simulink model "FSAC2021_V1_Running"  (R2014a)
settings: Solver=FixedStepDiscrete  StartTime=0.0  StopTime=inf  FixedStep=0.0005  RelTol=1e-3
model workspace (MAT data in the model file):
  MCOS : class17 (value not decoded)
  MCOS : class17 (value not decoded)
  MCOS : class17 (value not decoded)
  MCOS : class17 (value not decoded)
  MCOS : class17 (value not decoded)
  MCOS : class17 (value not decoded)
  MCOS : class17 (value not decoded)
  MCOS : class17 (value not decoded)
  MCOS : class17 (value not decoded)
  MCOS : class17 (value not decoded)
  MCOS : class17 (value not decoded)
  MCOS : class17 (value not decoded)
  MCOS : class17 (value not decoded)
  MCOS : class17 (value not decoded)
  MCOS : class17 (value not decoded)
  MCOS : class17 (value not decoded)
  MCOS : class17 (value not decoded)
  MCOS : class17 (value not decoded)
  MCOS : class17 (value not decoded)
  BUZZER_START = 1
  MCOS : class17 (value not decoded)
  MCOS : class17 (value not decoded)
  MCOS : class17 (value not decoded)
  MCOS : class17 (value not decoded)
  MCOS : class17 (value not decoded)
  MCOS : class17 (value not decoded)
  MCOS : class17 (value not decoded)
  MCOS : class17 (value not decoded)
  MCOS : class17 (value not decoded)
  MCOS : class17 (value not decoded)
  MCOS : class17 (value not decoded)
  MCOS : class17 (value not decoded)
  MCOS : class17 (value not decoded)
  MCOS : class17 (value not decoded)
  MCOS : class17 (value not decoded)
  MCOS : class17 (value not decoded)
  MCOS : class17 (value not decoded)
  MCOS : class17 (value not decoded)
  MCOS : class17 (value not decoded)
  MCOS : class17 (value not decoded)
  MCOS : class17 (value not decoded)
  MCOS : class17 (value not decoded)
  MCOS : class17 (value not decoded)
  MCOS : class17 (value not decoded)
  MCOS : class17 (value not decoded)
  MCOS : class17 (value not decoded)
  MCOS : class17 (value not decoded)
  MCOS : class17 (value not decoded)
  MCOS : class17 (value not decoded)
  MCOS : class17 (value not decoded)
  MCOS : class17 (value not decoded)
  MCOS : class17 (value not decoded)
  MCOS : class17 (value not decoded)
  MCOS : class17 (value not decoded)
  MCOS : class17 (value not decoded)
  MCOS : class17 (value not decoded)
  MCOS : class17 (value not decoded)
  MCOS : class17 (value not decoded)
  Brake = 11
  MCOS : class17 (value not decoded)
  MCOS : class17 (value not decoded)
  MCOS : class17 (value not decoded)
  MCOS : class17 (value not decoded)
  MCOS : class17 (value not decoded)
  MCOS : class17 (value not decoded)
  MCOS : class17 (value not decoded)
  MCOS : class17 (value not decoded)
  Sensor_Acc_b = 101.85
  Sensor_Acc_k = -0.0185
  Str_Sen_Orig_Angle = -341
  MCOS : class17 (value not decoded)
  Tire_D = 0.47
  T = 0.05
libraries: simulink x402, ec55xxlib x134
(part 7 of 17)

== system FSAC2021_V1_Running/VCU_CAN_Read/PCANB(BMS、DRIVE_MOTOR)/BMS_HCU_MAXT1 ==
  input : Inport
  function : TriggerPort  TriggerType=function-call
  CoolingCtl_Ad : Sum
  CoolingCtl_Convert : DataTypeConversion  OutDataTypeStr=uint32
  CoolingCtl_F : Gain
  CoolingCtl_L : simulink/Logic and Bit Operations/Bitwise Operator  logicop=AND  UseBitMask=on  BitMask=255  BitMaskRealWorld=Stored Integer
  CoolingCtl_O : Constant  Value=0  OutDataTypeStr=single
  CoolingCtl_S : ArithShift
  CoolingCtl_Sub : Subsystem
  CoolingCtl_sat : Saturate  UpperLimit=1  LowerLimit=0
  CoolingCtlcv : DataTypeConversion
  Demux : Demux  Outputs=8
  HeatingCtl_Ad : Sum
  HeatingCtl_Convert : DataTypeConversion  OutDataTypeStr=uint32
  HeatingCtl_F : Gain
  HeatingCtl_L : simulink/Logic and Bit Operations/Bitwise Operator  logicop=AND  UseBitMask=on  BitMask=255  BitMaskRealWorld=Stored Integer
  HeatingCtl_O : Constant  Value=0  OutDataTypeStr=single
  HeatingCtl_S : ArithShift
  HeatingCtl_Sub : Subsystem
  HeatingCtl_sat : Saturate  UpperLimit=1  LowerLimit=0
  HeatingCtlcv : DataTypeConversion
  MaxTempNo_Ad : Sum
  MaxTempNo_Convert : DataTypeConversion  OutDataTypeStr=uint32
  MaxTempNo_F : Gain
  MaxTempNo_L : simulink/Logic and Bit Operations/Bitwise Operator  logicop=AND  UseBitMask=on  BitMask=255  BitMaskRealWorld=Stored Integer
  MaxTempNo_O : Constant  Value=0  OutDataTypeStr=single
  MaxTempNo_S : ArithShift
  MaxTempNo_Sub : Subsystem
  MaxTempNo_sat : Saturate  UpperLimit=255  LowerLimit=0
  MaxTempNocv : DataTypeConversion
  MaxTemp_Ad : Sum
  MaxTemp_Convert : DataTypeConversion  OutDataTypeStr=uint32
  MaxTemp_F : Gain
  MaxTemp_L : simulink/Logic and Bit Operations/Bitwise Operator  logicop=AND  UseBitMask=on  BitMask=255  BitMaskRealWorld=Stored Integer
  MaxTemp_O : Constant  Value=-40  OutDataTypeStr=single
  MaxTemp_S : ArithShift
  MaxTemp_Sub : Subsystem
  MaxTemp_sat : Saturate  UpperLimit=120  LowerLimit=-40
  MaxTempcv : DataTypeConversion
  MinTempNo_Ad : Sum
  MinTempNo_Convert : DataTypeConversion  OutDataTypeStr=uint32
  MinTempNo_F : Gain
  MinTempNo_L : simulink/Logic and Bit Operations/Bitwise Operator  logicop=AND  UseBitMask=on  BitMask=255  BitMaskRealWorld=Stored Integer
  MinTempNo_O : Constant  Value=0  OutDataTypeStr=single
  MinTempNo_S : ArithShift
  MinTempNo_Sub : Subsystem
  MinTempNo_sat : Saturate  UpperLimit=255  LowerLimit=0
  MinTempNocv : DataTypeConversion
  MinTemp_Ad : Sum
  MinTemp_Convert : DataTypeConversion  OutDataTypeStr=uint32
  MinTemp_F : Gain
  MinTemp_L : simulink/Logic and Bit Operations/Bitwise Operator  logicop=AND  UseBitMask=on  BitMask=255  BitMaskRealWorld=Stored Integer
  MinTemp_O : Constant  Value=-40  OutDataTypeStr=single
  MinTemp_S : ArithShift
  MinTemp_Sub : Subsystem
  MinTemp_sat : Saturate  UpperLimit=120  LowerLimit=-40
  MinTempcv : DataTypeConversion
  HeatingCtl_Out : Outport
  CoolingCtl_Out : Outport  Port=2
  MinTempNo_Out : Outport  Port=3
  MaxTempNo_Out : Outport  Port=4
  MinTemp_Out : Outport  Port=5
  MaxTemp_Out : Outport  Port=6
  wires:
  HeatingCtl_F/1 -> HeatingCtl_Ad/1
  HeatingCtl_O/1 -> HeatingCtl_Ad/2
  HeatingCtl_Ad/1 -> HeatingCtl_sat/1
  HeatingCtl_sat/1 -> HeatingCtl_Out/1
  Demux/6 -> HeatingCtl_Sub/1(In1)
  HeatingCtl_Sub/1(Out1) -> HeatingCtl_Convert/1
  HeatingCtl_Convert/1 -> HeatingCtl_L/1
  HeatingCtl_L/1 -> HeatingCtl_S/1
  HeatingCtl_S/1 -> HeatingCtlcv/1
  HeatingCtlcv/1 -> HeatingCtl_F/1
  CoolingCtl_F/1 -> CoolingCtl_Ad/1
  CoolingCtl_O/1 -> CoolingCtl_Ad/2
  CoolingCtl_Ad/1 -> CoolingCtl_sat/1
  CoolingCtl_sat/1 -> CoolingCtl_Out/1
  Demux/5 -> CoolingCtl_Sub/1(In1)
  CoolingCtl_Sub/1(Out1) -> CoolingCtl_Convert/1
  CoolingCtl_Convert/1 -> CoolingCtl_L/1
  CoolingCtl_L/1 -> CoolingCtl_S/1
  CoolingCtl_S/1 -> CoolingCtlcv/1
  CoolingCtlcv/1 -> CoolingCtl_F/1
  MinTempNo_F/1 -> MinTempNo_Ad/1
  MinTempNo_O/1 -> MinTempNo_Ad/2
  MinTempNo_Ad/1 -> MinTempNo_sat/1
  MinTempNo_sat/1 -> MinTempNo_Out/1
  Demux/4 -> MinTempNo_Sub/1(In1)
  MinTempNo_Sub/1(Out1) -> MinTempNo_Convert/1
  MinTempNo_Convert/1 -> MinTempNo_L/1
  MinTempNo_L/1 -> MinTempNo_S/1
  MinTempNo_S/1 -> MinTempNocv/1
  MinTempNocv/1 -> MinTempNo_F/1
  MaxTempNo_F/1 -> MaxTempNo_Ad/1
  MaxTempNo_O/1 -> MaxTempNo_Ad/2
  MaxTempNo_Ad/1 -> MaxTempNo_sat/1
  MaxTempNo_sat/1 -> MaxTempNo_Out/1
  Demux/3 -> MaxTempNo_Sub/1(In1)
  MaxTempNo_Sub/1(Out1) -> MaxTempNo_Convert/1
  MaxTempNo_Convert/1 -> MaxTempNo_L/1
  MaxTempNo_L/1 -> MaxTempNo_S/1
  MaxTempNo_S/1 -> MaxTempNocv/1
  MaxTempNocv/1 -> MaxTempNo_F/1
  MinTemp_F/1 -> MinTemp_Ad/1
  MinTemp_O/1 -> MinTemp_Ad/2
  MinTemp_Ad/1 -> MinTemp_sat/1
  MinTemp_sat/1 -> MinTemp_Out/1
  Demux/2 -> MinTemp_Sub/1(In1)
  MinTemp_Sub/1(Out1) -> MinTemp_Convert/1
  MinTemp_Convert/1 -> MinTemp_L/1
  MinTemp_L/1 -> MinTemp_S/1
  MinTemp_S/1 -> MinTempcv/1
  MinTempcv/1 -> MinTemp_F/1
  MaxTemp_F/1 -> MaxTemp_Ad/1
  MaxTemp_O/1 -> MaxTemp_Ad/2
  MaxTemp_Ad/1 -> MaxTemp_sat/1
  MaxTemp_sat/1 -> MaxTemp_Out/1
  Demux/1 -> MaxTemp_Sub/1(In1)
  MaxTemp_Sub/1(Out1) -> MaxTemp_Convert/1
  MaxTemp_Convert/1 -> MaxTemp_L/1
  MaxTemp_L/1 -> MaxTemp_S/1
  MaxTemp_S/1 -> MaxTempcv/1
  MaxTempcv/1 -> MaxTemp_F/1
  input/1 -> Demux/1

== system FSAC2021_V1_Running/VCU_CAN_Read/PCANB(BMS、DRIVE_MOTOR)/BMS_HCU_MAXV  ==
  In1 : Inport
  function : TriggerPort  TriggerType=function-call
  BMS_HCU_MAXV : Subsystem
  Data Type Conversion{8..11} (4 alike) : DataTypeConversion  OutDataTypeStr=uint16
  MaxCellVoltNo_Out : Outport
  MinCellVoltNo_Out : Outport  Port=2
  MinCellVolt_Out : Outport  Port=3
  MaxCellVolt_Out : Outport  Port=4
  wires:
  BMS_HCU_MAXV/3(MinCellVolt_Out) -> Data Type Conversion10/1
  BMS_HCU_MAXV/4(MaxCellVolt_Out) -> Data Type Conversion11/1
  BMS_HCU_MAXV/1(MaxCellVoltNo_Out) -> Data Type Conversion8/1
  BMS_HCU_MAXV/2(MinCellVoltNo_Out) -> Data Type Conversion9/1
  Data Type Conversion8/1 -> MaxCellVoltNo_Out/1
  Data Type Conversion9/1 -> MinCellVoltNo_Out/1
  Data Type Conversion10/1 -> MinCellVolt_Out/1
  Data Type Conversion11/1 -> MaxCellVolt_Out/1
  In1/1 -> BMS_HCU_MAXV/1(input)

== system FSAC2021_V1_Running/VCU_CAN_Read/PCANB(BMS、DRIVE_MOTOR)/BMS_HCU_POWER  ==
  In1 : Inport
  function : TriggerPort  TriggerType=function-call
  BMS_HCU_POWER : Subsystem
  Data Type Conversion{74..77} (4 alike) : DataTypeConversion  OutDataTypeStr=double
  MaxDisPowerLimit_Out : Outport
  MaxChrPowerLimit_Out : Outport  Port=2
  MaxDisCurtLimit_Out : Outport  Port=3
  MaxChrCurtLimit_Out : Outport  Port=4
  wires:
  Data Type Conversion75/1 -> MaxChrPowerLimit_Out/1
  Data Type Conversion74/1 -> MaxDisPowerLimit_Out/1
  Data Type Conversion76/1 -> MaxDisCurtLimit_Out/1
  Data Type Conversion77/1 -> MaxChrCurtLimit_Out/1
  BMS_HCU_POWER/2(MaxChrPowerLimit_Out) -> Data Type Conversion75/1
  BMS_HCU_POWER/3(MaxDisCurtLimit_Out) -> Data Type Conversion76/1
  BMS_HCU_POWER/4(MaxChrCurtLimit_Out) -> Data Type Conversion77/1
  BMS_HCU_POWER/1(MaxDisPowerLimit_Out) -> Data Type Conversion74/1
  In1/1 -> BMS_HCU_POWER/1(input)

== system FSAC2021_V1_Running/VCU_CAN_Read/PCANB(BMS、DRIVE_MOTOR)/BMS_RELAY  ==
  In1 : Inport
  function : TriggerPort  TriggerType=function-call
  BMS_HCU_RELAY : Subsystem
  Data Type Conversion{63,66..73} (9 alike) : DataTypeConversion  OutDataTypeStr=uint8
  Data Type Conversion64 : DataTypeConversion  OutDataTypeStr=double
  Data Type Conversion65 : DataTypeConversion  OutDataTypeStr=double
  offChrRlyStr_Out : Outport
  ChrReqCurr_Out : Outport  Port=2
  ChrReqVolt_Out : Outport  Port=3
  chrONCC_Out : Outport  Port=4
  chrOFFCC2_Out : Outport  Port=5
  ChrCommunication_Out : Outport  Port=6
  ChrState_Out : Outport  Port=7
  OnChrRlyStr_Out : Outport  Port=8
  PreRlyStr_Out : Outport  Port=9
  NegRlyStr_Out : Outport  Port=10
  PosRlyStr_Out : Outport  Port=11
  wires:
  Data Type Conversion67/1 -> chrOFFCC2_Out/1
  Data Type Conversion63/1 -> offChrRlyStr_Out/1
  Data Type Conversion64/1 -> ChrReqCurr_Out/1
  Data Type Conversion69/1 -> ChrState_Out/1
  Data Type Conversion71/1 -> PreRlyStr_Out/1
  Data Type Conversion65/1 -> ChrReqVolt_Out/1
  Data Type Conversion73/1 -> PosRlyStr_Out/1
  Data Type Conversion72/1 -> NegRlyStr_Out/1
  Data Type Conversion66/1 -> chrONCC_Out/1
  Data Type Conversion68/1 -> ChrCommunication_Out/1
  Data Type Conversion70/1 -> OnChrRlyStr_Out/1
  BMS_HCU_RELAY/1(offChrRlyStr_Out) -> Data Type Conversion63/1
  BMS_HCU_RELAY/2(ChrReqCurr_Out) -> Data Type Conversion64/1
  BMS_HCU_RELAY/4(chrONCC_Out) -> Data Type Conversion66/1
  BMS_HCU_RELAY/9(PreRlyStr_Out) -> Data Type Conversion71/1
  BMS_HCU_RELAY/11(PosRlyStr_Out) -> Data Type Conversion73/1
  BMS_HCU_RELAY/8(OnChrRlyStr_Out) -> Data Type Conversion70/1
  BMS_HCU_RELAY/5(chrOFFCC2_Out) -> Data Type Conversion67/1
  BMS_HCU_RELAY/10(NegRlyStr_Out) -> Data Type Conversion72/1
  BMS_HCU_RELAY/6(ChrCommunication_Out) -> Data Type Conversion68/1
  BMS_HCU_RELAY/3(ChrReqVolt_Out) -> Data Type Conversion65/1
  BMS_HCU_RELAY/7(ChrState_Out) -> Data Type Conversion69/1
  In1/1 -> BMS_HCU_RELAY/1(input)

== system FSAC2021_V1_Running/VCU_CAN_Read/PCANB(BMS、DRIVE_MOTOR)/MOTOR_CURRENT_SPEED ==
  input : Inport
  function : TriggerPort  TriggerType=function-call
  Demux : Demux  Outputs=2
  Motor_Currt_Speed_Ad : Sum
  Motor_Currt_Speed_Convert : DataTypeConversion  OutDataTypeStr=uint32
  Motor_Currt_Speed_F : Gain
  Motor_Currt_Speed_L : simulink/Logic and Bit Operations/Bitwise Operator  logicop=AND  UseBitMask=on  BitMask=65535  BitMaskRealWorld=Stored Integer
  Motor_Currt_Speed_O : Constant  Value=0  OutDataTypeStr=single
  Motor_Currt_Speed_S : ArithShift
  Motor_Currt_Speed_Sub : Subsystem
  Motor_Currt_Speed_sat : Saturate  UpperLimit=2500  LowerLimit=0
  Motor_Currt_Speedcv : DataTypeConversion
  Motor_Currt_Speedinput2_Ad : Sum
  Motor_Currt_Speedinput2_C : Constant  Value=256
  Motor_Currt_Speedinput2_P : Product
  Motor_Currt_Speed_Out : Outport
  wires:
  Motor_Currt_Speed_F/1 -> Motor_Currt_Speed_Ad/1
  Motor_Currt_Speed_O/1 -> Motor_Currt_Speed_Ad/2
  Motor_Currt_Speed_Ad/1 -> Motor_Currt_Speed_sat/1
  Motor_Currt_Speed_sat/1 -> Motor_Currt_Speed_Out/1
  Demux/2 -> Motor_Currt_Speedinput2_P/1
  Motor_Currt_Speedinput2_C/1 -> Motor_Currt_Speedinput2_P/2
  Motor_Currt_Speedinput2_P/1 -> Motor_Currt_Speedinput2_Ad/1
  Demux/1 -> Motor_Currt_Speedinput2_Ad/2
  Motor_Currt_Speedinput2_Ad/1 -> Motor_Currt_Speed_Sub/1(In1)
  Motor_Currt_Speed_Sub/1(Out1) -> Motor_Currt_Speed_Convert/1
  Motor_Currt_Speed_Convert/1 -> Motor_Currt_Speed_L/1
  Motor_Currt_Speed_L/1 -> Motor_Currt_Speed_S/1
  Motor_Currt_Speed_S/1 -> Motor_Currt_Speedcv/1
  Motor_Currt_Speedcv/1 -> Motor_Currt_Speed_F/1
  input/1 -> Demux/1

== system FSAC2021_V1_Running/VCU_CAN_Read/Subsystem/BMS_HCU_INFO  ==
  In1 : Inport
  function : TriggerPort  TriggerType=function-call
  BMS_HCU_INFO : Subsystem
  Data Type Conversion{78..82} (5 alike) : DataTypeConversion  OutDataTypeStr=uint8
  Data Type Conversion83 : DataTypeConversion  OutDataTypeStr=double
  Data Type Conversion84 : DataTypeConversion  OutDataTypeStr=double
  BatLife_Out : Outport
  BatAlmLv_Out : Outport  Port=2
  BatState_Out : Outport  Port=3
  BatSoh_Out : Outport  Port=4
  BatSoc_Out : Outport  Port=5
  BatCurrent_Out : Outport  Port=6
  BatVoltage_Out : Outport  Port=7
  wires:
  Data Type Conversion79/1 -> BatAlmLv_Out/1
  Data Type Conversion80/1 -> BatState_Out/1
  Data Type Conversion84/1 -> BatVoltage_Out/1
  Data Type Conversion82/1 -> BatSoc_Out/1
  Data Type Conversion78/1 -> BatLife_Out/1
  Data Type Conversion81/1 -> BatSoh_Out/1
  Data Type Conversion83/1 -> BatCurrent_Out/1
  BMS_HCU_INFO/3(BatState_Out) -> Data Type Conversion80/1
  BMS_HCU_INFO/6(BatCurrent_Out) -> Data Type Conversion83/1
  BMS_HCU_INFO/4(BatSoh_Out) -> Data Type Conversion81/1
  BMS_HCU_INFO/5(BatSoc_Out) -> Data Type Conversion82/1
  BMS_HCU_INFO/7(BatVoltage_Out) -> Data Type Conversion84/1
  BMS_HCU_INFO/1(BatLife_Out) -> Data Type Conversion78/1
  BMS_HCU_INFO/2(BatAlmLv_Out) -> Data Type Conversion79/1
  In1/1 -> BMS_HCU_INFO/1(input)

== system FSAC2021_V1_Running/VCU_CAN_Read/Subsystem1/HEARTBEAT  ==
  In1 : Inport
  function : TriggerPort  TriggerType=function-call
  Data Type Conversion21 : DataTypeConversion  OutDataTypeStr=uint8
  MOTEC_HEARTBEAT : Subsystem
  Heartbeat_info_Out : Outport
  wires:
  MOTEC_HEARTBEAT/1(Heartbeat_info_Out) -> Data Type Conversion21/1
  Data Type Conversion21/1 -> Heartbeat_info_Out/1
  In1/1 -> MOTEC_HEARTBEAT/1(input)

== system FSAC2021_V1_Running/VCU_CAN_Read/Subsystem2/MOTEC_STATUS  ==
  In1 : Inport
  function : TriggerPort  TriggerType=function-call
  Data Type Conversion{13,15..20,106..107} (9 alike) : DataTypeConversion  OutDataTypeStr=uint8
  MOTEC_STATUS : Subsystem
  Fault_Out : Outport
  Operation_Enabled_Out : Outport  Port=2
  Quick_Stop_Out : Outport  Port=3
  Ready_Switch_On_Out : Outport  Port=4
  Switch_On_Disabled_Out : Outport  Port=5
  Swtiched_On_Out : Outport  Port=6
  Target_Reached_Out : Outport  Port=7
  Voltage_Enabled_Out : Outport  Port=8
  Warning_Out : Outport  Port=9
  wires:
  In1/1 -> MOTEC_STATUS/1(input)
  MOTEC_STATUS/3(Quick_Stop_Out) -> Data Type Conversion16/1
  MOTEC_STATUS/4(Ready_Switch_On_Out) -> Data Type Conversion17/1
  MOTEC_STATUS/5(Switch_On_Disabled_Out) -> Data Type Conversion18/1
  MOTEC_STATUS/6(Swtiched_On_Out) -> Data Type Conversion19/1
  MOTEC_STATUS/1(Fault_Out) -> Data Type Conversion13/1
  MOTEC_STATUS/2(Operation_Enabled_Out) -> Data Type Conversion15/1
  Data Type Conversion15/1 -> Operation_Enabled_Out/1
  Data Type Conversion17/1 -> Ready_Switch_On_Out/1
  Data Type Conversion20/1 -> Target_Reached_Out/1
  Data Type Conversion19/1 -> Swtiched_On_Out/1
  Data Type Conversion16/1 -> Quick_Stop_Out/1
  Data Type Conversion18/1 -> Switch_On_Disabled_Out/1
  MOTEC_STATUS/8(Voltage_Enabled_Out) -> Data Type Conversion106/1
  Data Type Conversion107/1 -> Warning_Out/1
  MOTEC_STATUS/7(Target_Reached_Out) -> Data Type Conversion20/1
  MOTEC_STATUS/9(Warning_Out) -> Data Type Conversion107/1
  Data Type Conversion106/1 -> Voltage_Enabled_Out/1
  Data Type Conversion13/1 -> Fault_Out/1

== system FSAC2021_V1_Running/CAN_SEND/(BRK、STR、DRIVER)/BCU_MTR_MOVE_AB/Brake_mtr_goalpos ==
  Brake_mtr_goalpos : Inport
  Brake_mtr_goalposABS : Abs
  Brake_mtr_goalposBitCov : DataTypeConversion  OutDataTypeStr=uint32
  Brake_mtr_goalposBitCov1 : DataTypeConversion  OutDataTypeStr=uint32
  Brake_mtr_goalposBitCov2 : DataTypeConversion  OutDataTypeStr=uint8
  Brake_mtr_goalposCOV : DataTypeConversion  OutDataTypeStr=uint8
  Brake_mtr_goalposCOV1 : DataTypeConversion  OutDataTypeStr=uint8
  Brake_mtr_goalposCOV2 : DataTypeConversion  OutDataTypeStr=uint8
  Brake_mtr_goalposCS : ArithShift  BitShiftNumber=-32
  Brake_mtr_goalposConS : Constant  OutDataTypeStr=single
  Brake_mtr_goalposCosR : Constant  Value=0  OutDataTypeStr=uint8
  Brake_mtr_goalposROP : RelationalOperator  Operator=<  OutDataTypeStr=boolean
  Brake_mtr_goalposRon : Rounding  Operator=round
  Brake_mtr_goalposSW : Switch  Criteria=u2 ~= 0
  Brake_mtr_goalpos_1sat : Saturate  UpperLimit=4294967295  LowerLimit=0
  Brake_mtr_goalpos_And : simulink/Logic and Bit Operations/Bitwise Operator  logicop=AND  UseBitMask=off  NumInputPorts=2  BitMask=bin2dec('11011001')  BitMaskRealWorld=Stored Integer
  Brake_mtr_goalpos_And1 : simulink/Logic and Bit Operations/Bitwise Operator  logicop=AND  UseBitMask=off  NumInputPorts=2  BitMask=bin2dec('11011001')  BitMaskRealWorld=Stored Integer
  Brake_mtr_goalpos_And1_C : Constant  Value=65535
  Brake_mtr_goalpos_And2 : simulink/Logic and Bit Operations/Bitwise Operator  logicop=AND  UseBitMask=off  NumInputPorts=2  BitMask=bin2dec('11011001')  BitMaskRealWorld=Stored Integer
  Brake_mtr_goalpos_And2_C : Constant  Value=255  OutDataTypeStr=uint32
  Brake_mtr_goalpos_And_C : Constant  Value=16777215
  Brake_mtr_goalpos_Convert : DataTypeConversion  OutDataTypeStr=uint32
  Brake_mtr_goalpos_D{,1..3} (4 alike) : Product  Inputs=*/
  Brake_mtr_goalpos_F : Constant  OutDataTypeStr=single
  Brake_mtr_goalpos_L : simulink/Logic and Bit Operations/Bitwise Operator  logicop=AND  UseBitMask=on  BitMask=4294967295  BitMaskRealWorld=Stored Integer
  Brake_mtr_goalpos_O : Constant  Value=0  OutDataTypeStr=single
  Brake_mtr_goalpos_S : ArithShift
  Brake_mtr_goalpos_sat : Saturate  UpperLimit=2147483647  LowerLimit=-2147483648
  Brake_mtr_goalpos_st : Sum  Inputs=+-
  Brake_mtr_goalpos_swtsig : Switch  Criteria=u2 ~= 0
  Brake_mtr_goalposoutput2_C : Constant  Value=256
  Brake_mtr_goalposoutput3_C : Constant  Value=65536
  Brake_mtr_goalposoutput4_C : Constant  Value=16777216
  Brake_mtr_goalpossatAbs : Saturate  UpperLimit=2147483647  LowerLimit=0
  Brake_mtr_goalpossubcon : Sum  Inputs=+-
  output1 : Outport
  output2 : Outport  Port=2
  output3 : Outport  Port=3
  output4 : Outport  Port=4
  wires:
  Brake_mtr_goalpos/1 -> Brake_mtr_goalpos_sat/1
  Brake_mtr_goalpos_sat/1 -> Brake_mtr_goalpos_st/1
  Brake_mtr_goalpos_O/1 -> Brake_mtr_goalpos_st/2
  Brake_mtr_goalpos_st/1 -> Brake_mtr_goalpos_D/1
  Brake_mtr_goalpos_F/1 -> Brake_mtr_goalpos_D/2
  Brake_mtr_goalpos_D/1 -> Brake_mtr_goalposRon/1
  Brake_mtr_goalpossatAbs/1 -> Brake_mtr_goalpos_swtsig/1, Brake_mtr_goalposSW/3
  Brake_mtr_goalposROP/1 -> Brake_mtr_goalpos_swtsig/2, Brake_mtr_goalposSW/2
  Brake_mtr_goalposRon/1 -> Brake_mtr_goalposROP/1, Brake_mtr_goalposABS/1, Brake_mtr_goalpos_swtsig/3
  Brake_mtr_goalpos_swtsig/1 -> Brake_mtr_goalpossubcon/2
  Brake_mtr_goalposCosR/1 -> Brake_mtr_goalposROP/2
  Brake_mtr_goalposConS/1 -> Brake_mtr_goalposCS/1
  Brake_mtr_goalposCS/1 -> Brake_mtr_goalpossubcon/1
  Brake_mtr_goalposABS/1 -> Brake_mtr_goalpossatAbs/1
  Brake_mtr_goalpossubcon/1 -> Brake_mtr_goalposSW/1
  Brake_mtr_goalposSW/1 -> Brake_mtr_goalpos_S/1
  Brake_mtr_goalpos_S/1 -> Brake_mtr_goalpos_1sat/1
  Brake_mtr_goalpos_1sat/1 -> Brake_mtr_goalpos_Convert/1
  Brake_mtr_goalpos_Convert/1 -> Brake_mtr_goalpos_L/1
  Brake_mtr_goalpos_L/1 -> Brake_mtr_goalpos_And1/1, Brake_mtr_goalpos_And2/1, Brake_mtr_goalpos_And/1, Brake_mtr_goalpos_D1/1
  Brake_mtr_goalposoutput4_C/1 -> Brake_mtr_goalpos_D1/2
  Brake_mtr_goalpos_D1/1 -> Brake_mtr_goalposCOV/1
  Brake_mtr_goalposCOV/1 -> output1/1
  Brake_mtr_goalpos_And_C/1 -> Brake_mtr_goalposBitCov/1
  Brake_mtr_goalposBitCov/1 -> Brake_mtr_goalpos_And/2
  Brake_mtr_goalpos_And/1 -> Brake_mtr_goalpos_D2/1
  Brake_mtr_goalposoutput3_C/1 -> Brake_mtr_goalpos_D2/2
  Brake_mtr_goalpos_D2/1 -> Brake_mtr_goalposCOV1/1
  Brake_mtr_goalposCOV1/1 -> output2/1
  Brake_mtr_goalpos_And1_C/1 -> Brake_mtr_goalposBitCov1/1
  Brake_mtr_goalposBitCov1/1 -> Brake_mtr_goalpos_And1/2
  Brake_mtr_goalpos_And1/1 -> Brake_mtr_goalpos_D3/1
  Brake_mtr_goalposoutput2_C/1 -> Brake_mtr_goalpos_D3/2
  Brake_mtr_goalpos_D3/1 -> Brake_mtr_goalposCOV2/1
  Brake_mtr_goalposCOV2/1 -> output3/1
  Brake_mtr_goalpos_And2_C/1 -> Brake_mtr_goalpos_And2/2
  Brake_mtr_goalpos_And2/1 -> Brake_mtr_goalposBitCov2/1
  Brake_mtr_goalposBitCov2/1 -> output4/1

== system FSAC2021_V1_Running/CAN_SEND/(BRK、STR、DRIVER)/BCU_STATUS_READ/status_reg_addr_start ==
  status_reg_addr_start : Inport
  status_reg_addr_startRon : Rounding  Operator=round
  status_reg_addr_start_1sat : Saturate  UpperLimit=255  LowerLimit=0
  status_reg_addr_start_Convert : DataTypeConversion  OutDataTypeStr=uint8
  status_reg_addr_start_Convert1 : DataTypeConversion  OutDataTypeStr=uint32
  status_reg_addr_start_D : Product  Inputs=*/
  status_reg_addr_start_F : Constant  OutDataTypeStr=single
  status_reg_addr_start_L : simulink/Logic and Bit Operations/Bitwise Operator  logicop=AND  UseBitMask=on  BitMask=255  BitMaskRealWorld=Stored Integer
  status_reg_addr_start_O : Constant  Value=0  OutDataTypeStr=single
  status_reg_addr_start_S : ArithShift
  status_reg_addr_start_sat : Saturate  UpperLimit=255  LowerLimit=0
  status_reg_addr_start_st : Sum  Inputs=+-
  output1 : Outport
  wires:
  status_reg_addr_start/1 -> status_reg_addr_start_sat/1
  status_reg_addr_start_sat/1 -> status_reg_addr_start_st/1
  status_reg_addr_start_O/1 -> status_reg_addr_start_st/2
  status_reg_addr_start_st/1 -> status_reg_addr_start_D/1
  status_reg_addr_start_F/1 -> status_reg_addr_start_D/2
  status_reg_addr_start_D/1 -> status_reg_addr_startRon/1
  status_reg_addr_startRon/1 -> status_reg_addr_start_S/1
  status_reg_addr_start_S/1 -> status_reg_addr_start_1sat/1
  status_reg_addr_start_1sat/1 -> status_reg_addr_start_Convert1/1
  status_reg_addr_start_Convert1/1 -> status_reg_addr_start_L/1
  status_reg_addr_start_L/1 -> status_reg_addr_start_Convert/1
  status_reg_addr_start_Convert/1 -> output1/1

== system FSAC2021_V1_Running/CAN_SEND/(BRK、STR、DRIVER)/BCU_STATUS_READ/status_reg_num ==
  status_reg_num : Inport
  status_reg_numRon : Rounding  Operator=round
  status_reg_num_1sat : Saturate  UpperLimit=255  LowerLimit=0
  status_reg_num_Convert : DataTypeConversion  OutDataTypeStr=uint8
  status_reg_num_Convert1 : DataTypeConversion  OutDataTypeStr=uint32
  status_reg_num_D : Product  Inputs=*/
  status_reg_num_F : Constant  OutDataTypeStr=single
  status_reg_num_L : simulink/Logic and Bit Operations/Bitwise Operator  logicop=AND  UseBitMask=on  BitMask=255  BitMaskRealWorld=Stored Integer
  status_reg_num_O : Constant  Value=0  OutDataTypeStr=single
  status_reg_num_S : ArithShift
  status_reg_num_sat : Saturate  UpperLimit=255  LowerLimit=0
  status_reg_num_st : Sum  Inputs=+-
  output2 : Outport
  wires:
  status_reg_num/1 -> status_reg_num_sat/1
  status_reg_num_sat/1 -> status_reg_num_st/1
  status_reg_num_O/1 -> status_reg_num_st/2
  status_reg_num_st/1 -> status_reg_num_D/1
  status_reg_num_F/1 -> status_reg_num_D/2
  status_reg_num_D/1 -> status_reg_numRon/1
  status_reg_numRon/1 -> status_reg_num_S/1
  status_reg_num_S/1 -> status_reg_num_1sat/1
  status_reg_num_1sat/1 -> status_reg_num_Convert1/1
  status_reg_num_Convert1/1 -> status_reg_num_L/1
  status_reg_num_L/1 -> status_reg_num_Convert/1
  status_reg_num_Convert/1 -> output2/1

== system FSAC2021_V1_Running/CAN_SEND/(BRK、STR、DRIVER)/MOTOR_SPEED_CONTROL/Drive_Speed_Control ==
  Drive_Speed_Control : Inport
  BitCov : DataTypeConversion  OutDataTypeStr=uint8
  Drive_Speed_ControlCOV : DataTypeConversion  OutDataTypeStr=uint8
  Drive_Speed_ControlRon : Rounding  Operator=round
  Drive_Speed_Control_1sat : Saturate  UpperLimit=65535  LowerLimit=0
  Drive_Speed_Control_And : simulink/Logic and Bit Operations/Bitwise Operator  logicop=AND  UseBitMask=off  NumInputPorts=2  BitMask=bin2dec('11011001')  BitMaskRealWorld=Stored Integer
  Drive_Speed_Control_And_C : Constant  Value=255  OutDataTypeStr=uint32
  Drive_Speed_Control_Convert : DataTypeConversion  OutDataTypeStr=uint32
  Drive_Speed_Control_D : Product  Inputs=*/
  Drive_Speed_Control_D1 : Product  Inputs=*/
  Drive_Speed_Control_F : Constant  OutDataTypeStr=single
  Drive_Speed_Control_L : simulink/Logic and Bit Operations/Bitwise Operator  logicop=AND  UseBitMask=on  BitMask=65535  BitMaskRealWorld=Stored Integer
  Drive_Speed_Control_O : Constant  Value=0  OutDataTypeStr=single
  Drive_Speed_Control_S : ArithShift
  Drive_Speed_Control_sat : Saturate  UpperLimit=1500  LowerLimit=0
  Drive_Speed_Control_st : Sum  Inputs=+-
  Drive_Speed_Controloutput2_C : Constant  Value=256
  output1 : Outport
  output2 : Outport  Port=2
  wires:
  Drive_Speed_Control/1 -> Drive_Speed_Control_sat/1
  Drive_Speed_Control_sat/1 -> Drive_Speed_Control_st/1
  Drive_Speed_Control_O/1 -> Drive_Speed_Control_st/2
  Drive_Speed_Control_st/1 -> Drive_Speed_Control_D/1
  Drive_Speed_Control_F/1 -> Drive_Speed_Control_D/2
  Drive_Speed_Control_D/1 -> Drive_Speed_ControlRon/1
  Drive_Speed_ControlRon/1 -> Drive_Speed_Control_S/1
  Drive_Speed_Control_S/1 -> Drive_Speed_Control_1sat/1
  Drive_Speed_Control_1sat/1 -> Drive_Speed_Control_Convert/1
  Drive_Speed_Control_Convert/1 -> Drive_Speed_Control_L/1
  Drive_Speed_Control_L/1 -> Drive_Speed_Control_D1/1, Drive_Speed_Control_And/1
  Drive_Speed_Controloutput2_C/1 -> Drive_Speed_Control_D1/2
  Drive_Speed_Control_D1/1 -> Drive_Speed_ControlCOV/1
  Drive_Speed_ControlCOV/1 -> output2/1
  Drive_Speed_Control_And_C/1 -> Drive_Speed_Control_And/2
  Drive_Speed_Control_And/1 -> BitCov/1
  BitCov/1 -> output1/1

== system FSAC2021_V1_Running/CAN_SEND/(BRK、STR、DRIVER)/To_AMI/Battery_Volt ==
  Battery_Volt : Inport
  Battery_VoltBitCov : DataTypeConversion  OutDataTypeStr=uint8
  Battery_VoltCOV : DataTypeConversion  OutDataTypeStr=uint8
  Battery_VoltRon : Rounding  Operator=round
  Battery_Volt_1sat : Saturate  UpperLimit=65535  LowerLimit=0
  Battery_Volt_And : simulink/Logic and Bit Operations/Bitwise Operator  logicop=AND  UseBitMask=off  NumInputPorts=2  BitMask=bin2dec('11011001')  BitMaskRealWorld=Stored Integer
  Battery_Volt_And_C : Constant  Value=255  OutDataTypeStr=uint32
  Battery_Volt_Convert : DataTypeConversion  OutDataTypeStr=uint32
  Battery_Volt_D : Product  Inputs=*/
  Battery_Volt_D1 : Product  Inputs=*/
  Battery_Volt_F : Constant  Value=0.1  OutDataTypeStr=single
  Battery_Volt_L : simulink/Logic and Bit Operations/Bitwise Operator  logicop=AND  UseBitMask=on  BitMask=65535  BitMaskRealWorld=Stored Integer
  Battery_Volt_O : Constant  Value=0  OutDataTypeStr=single
  Battery_Volt_S : ArithShift
  Battery_Volt_sat : Saturate  UpperLimit=6553.5  LowerLimit=0
  Battery_Volt_st : Sum  Inputs=+-
  Battery_Voltoutput5_C : Constant  Value=256
  output5 : Outport
  output6 : Outport  Port=2
  wires:
  Battery_Volt/1 -> Battery_Volt_sat/1
  Battery_Volt_sat/1 -> Battery_Volt_st/1
  Battery_Volt_O/1 -> Battery_Volt_st/2
  Battery_Volt_st/1 -> Battery_Volt_D/1
  Battery_Volt_F/1 -> Battery_Volt_D/2
  Battery_Volt_D/1 -> Battery_VoltRon/1
  Battery_VoltRon/1 -> Battery_Volt_S/1
  Battery_Volt_S/1 -> Battery_Volt_1sat/1
  Battery_Volt_1sat/1 -> Battery_Volt_Convert/1
  Battery_Volt_Convert/1 -> Battery_Volt_L/1
  Battery_Volt_L/1 -> Battery_Volt_D1/1, Battery_Volt_And/1
  Battery_Voltoutput5_C/1 -> Battery_Volt_D1/2
  Battery_Volt_D1/1 -> Battery_VoltCOV/1
  Battery_VoltCOV/1 -> output5/1
  Battery_Volt_And_C/1 -> Battery_Volt_And/2
  Battery_Volt_And/1 -> Battery_VoltBitCov/1
  Battery_VoltBitCov/1 -> output6/1

== system FSAC2021_V1_Running/CAN_SEND/(BRK、STR、DRIVER)/To_AMI/assi_status ==
  assi_status : Inport
  assi_statusRon : Rounding  Operator=round
  assi_status_1sat : Saturate  UpperLimit=255  LowerLimit=0
  assi_status_Convert : DataTypeConversion  OutDataTypeStr=uint8
  assi_status_Convert1 : DataTypeConversion  OutDataTypeStr=uint32
  assi_status_D : Product  Inputs=*/
  assi_status_F : Constant  OutDataTypeStr=single
  assi_status_L : simulink/Logic and Bit Operations/Bitwise Operator  logicop=AND  UseBitMask=on  BitMask=255  BitMaskRealWorld=Stored Integer
  assi_status_O : Constant  Value=0  OutDataTypeStr=single
  assi_status_S : ArithShift
  assi_status_sat : Saturate  UpperLimit=255  LowerLimit=0
  assi_status_st : Sum  Inputs=+-
  output4 : Outport
  wires:
  assi_status/1 -> assi_status_sat/1
  assi_status_sat/1 -> assi_status_st/1
  assi_status_O/1 -> assi_status_st/2
  assi_status_st/1 -> assi_status_D/1
  assi_status_F/1 -> assi_status_D/2
  assi_status_D/1 -> assi_statusRon/1
  assi_statusRon/1 -> assi_status_S/1
  assi_status_S/1 -> assi_status_1sat/1
  assi_status_1sat/1 -> assi_status_Convert1/1
  assi_status_Convert1/1 -> assi_status_L/1
  assi_status_L/1 -> assi_status_Convert/1
  assi_status_Convert/1 -> output4/1

== system FSAC2021_V1_Running/CAN_SEND/(BRK、STR、DRIVER)/To_AMI/mtr_rpm ==
  mtr_rpm : Inport
  mtr_rpmBitCov : DataTypeConversion  OutDataTypeStr=uint8
  mtr_rpmCOV : DataTypeConversion  OutDataTypeStr=uint8
  mtr_rpmRon : Rounding  Operator=round
  mtr_rpm_1sat : Saturate  UpperLimit=65535  LowerLimit=0
  mtr_rpm_And : simulink/Logic and Bit Operations/Bitwise Operator  logicop=AND  UseBitMask=off  NumInputPorts=2  BitMask=bin2dec('11011001')  BitMaskRealWorld=Stored Integer
  mtr_rpm_And_C : Constant  Value=255  OutDataTypeStr=uint32
  mtr_rpm_Convert : DataTypeConversion  OutDataTypeStr=uint32
  mtr_rpm_D : Product  Inputs=*/
  mtr_rpm_D1 : Product  Inputs=*/
  mtr_rpm_F : Constant  OutDataTypeStr=single
  mtr_rpm_L : simulink/Logic and Bit Operations/Bitwise Operator  logicop=AND  UseBitMask=on  BitMask=65535  BitMaskRealWorld=Stored Integer
  mtr_rpm_O : Constant  Value=0  OutDataTypeStr=single
  mtr_rpm_S : ArithShift
  mtr_rpm_sat : Saturate  UpperLimit=65535  LowerLimit=0
  mtr_rpm_st : Sum  Inputs=+-
  mtr_rpmoutput2_C : Constant  Value=256
  output2 : Outport
  output3 : Outport  Port=2
  wires:
  mtr_rpm/1 -> mtr_rpm_sat/1
  mtr_rpm_sat/1 -> mtr_rpm_st/1
  mtr_rpm_O/1 -> mtr_rpm_st/2
  mtr_rpm_st/1 -> mtr_rpm_D/1
  mtr_rpm_F/1 -> mtr_rpm_D/2
  mtr_rpm_D/1 -> mtr_rpmRon/1
  mtr_rpmRon/1 -> mtr_rpm_S/1
  mtr_rpm_S/1 -> mtr_rpm_1sat/1
  mtr_rpm_1sat/1 -> mtr_rpm_Convert/1
  mtr_rpm_Convert/1 -> mtr_rpm_L/1
  mtr_rpm_L/1 -> mtr_rpm_D1/1, mtr_rpm_And/1
  mtr_rpmoutput2_C/1 -> mtr_rpm_D1/2
  mtr_rpm_D1/1 -> mtr_rpmCOV/1
  mtr_rpmCOV/1 -> output2/1
  mtr_rpm_And_C/1 -> mtr_rpm_And/2
  mtr_rpm_And/1 -> mtr_rpmBitCov/1
  mtr_rpmBitCov/1 -> output3/1

== system FSAC2021_V1_Running/CAN_SEND/(BRK、STR、DRIVER)/To_AMI/vspd ==
  vspd : Inport
  vspdRon : Rounding  Operator=round
  vspd_1sat : Saturate  UpperLimit=255  LowerLimit=0
  vspd_Convert : DataTypeConversion  OutDataTypeStr=uint8
  vspd_Convert1 : DataTypeConversion  OutDataTypeStr=uint32
  vspd_D : Product  Inputs=*/
  vspd_F : Constant  OutDataTypeStr=single
  vspd_L : simulink/Logic and Bit Operations/Bitwise Operator  logicop=AND  UseBitMask=on  BitMask=255  BitMaskRealWorld=Stored Integer
  vspd_O : Constant  Value=0  OutDataTypeStr=single
  vspd_S : ArithShift
  vspd_sat : Saturate  UpperLimit=255  LowerLimit=0
  vspd_st : Sum  Inputs=+-
  output1 : Outport
  wires:
  vspd/1 -> vspd_sat/1
  vspd_sat/1 -> vspd_st/1
  vspd_O/1 -> vspd_st/2
  vspd_st/1 -> vspd_D/1
  vspd_F/1 -> vspd_D/2
  vspd_D/1 -> vspdRon/1
  vspdRon/1 -> vspd_S/1
  vspd_S/1 -> vspd_1sat/1
  vspd_1sat/1 -> vspd_Convert1/1
  vspd_Convert1/1 -> vspd_L/1
  vspd_L/1 -> vspd_Convert/1
  vspd_Convert/1 -> output1/1

== system FSAC2021_V1_Running/CAN_SEND/Subsystem1/Brk_Mtr_Enbale/BCU_MTR_ENABLE ==
  Constant : Constant  Value=0  OutDataTypeStr=uint8
  Mux : Mux  Inputs=8
  output : Outport
  wires:
  Mux/1 -> output/1
  Constant/1 -> Mux/1, Mux/2, Mux/3, Mux/8, Mux/7, Mux/6, Mux/5, Mux/4

== system FSAC2021_V1_Running/CAN_SEND/Subsystem1/MOTEC_CONTROL/Abs_or_Rel_Ctrl ==
  Abs_or_Rel_Ctrl : Inport
  Abs_or_Rel_CtrlRon : Rounding  Operator=round
  Abs_or_Rel_Ctrl_1sat : Saturate  UpperLimit=64  LowerLimit=0
  Abs_or_Rel_Ctrl_Convert : DataTypeConversion  OutDataTypeStr=uint8
  Abs_or_Rel_Ctrl_Convert1 : DataTypeConversion  OutDataTypeStr=uint32
  Abs_or_Rel_Ctrl_D : Product  Inputs=*/
  Abs_or_Rel_Ctrl_F : Constant  OutDataTypeStr=single
  Abs_or_Rel_Ctrl_L : simulink/Logic and Bit Operations/Bitwise Operator  logicop=AND  UseBitMask=on  BitMask=64  BitMaskRealWorld=Stored Integer
  Abs_or_Rel_Ctrl_O : Constant  Value=0  OutDataTypeStr=single
  Abs_or_Rel_Ctrl_S : ArithShift  BitShiftNumber=-6
  Abs_or_Rel_Ctrl_sat : Saturate  UpperLimit=1  LowerLimit=0
  Abs_or_Rel_Ctrl_st : Sum  Inputs=+-
  output1 : Outport
  wires:
  Abs_or_Rel_Ctrl/1 -> Abs_or_Rel_Ctrl_sat/1
  Abs_or_Rel_Ctrl_sat/1 -> Abs_or_Rel_Ctrl_st/1
  Abs_or_Rel_Ctrl_O/1 -> Abs_or_Rel_Ctrl_st/2
  Abs_or_Rel_Ctrl_st/1 -> Abs_or_Rel_Ctrl_D/1
  Abs_or_Rel_Ctrl_F/1 -> Abs_or_Rel_Ctrl_D/2
  Abs_or_Rel_Ctrl_D/1 -> Abs_or_Rel_CtrlRon/1
  Abs_or_Rel_CtrlRon/1 -> Abs_or_Rel_Ctrl_S/1
  Abs_or_Rel_Ctrl_S/1 -> Abs_or_Rel_Ctrl_1sat/1
  Abs_or_Rel_Ctrl_1sat/1 -> Abs_or_Rel_Ctrl_Convert1/1
  Abs_or_Rel_Ctrl_Convert1/1 -> Abs_or_Rel_Ctrl_L/1
  Abs_or_Rel_Ctrl_L/1 -> Abs_or_Rel_Ctrl_Convert/1
  Abs_or_Rel_Ctrl_Convert/1 -> output1/1

== system FSAC2021_V1_Running/CAN_SEND/Subsystem1/MOTEC_CONTROL/Enable_Operation_Ctrl ==
  Enable_Operation_Ctrl : Inport
  Enable_Operation_CtrlRon : Rounding  Operator=round
  Enable_Operation_Ctrl_1sat : Saturate  UpperLimit=8  LowerLimit=0
  Enable_Operation_Ctrl_Convert : DataTypeConversion  OutDataTypeStr=uint8
  Enable_Operation_Ctrl_Convert1 : DataTypeConversion  OutDataTypeStr=uint32
  Enable_Operation_Ctrl_D : Product  Inputs=*/
  Enable_Operation_Ctrl_F : Constant  OutDataTypeStr=single
  Enable_Operation_Ctrl_L : simulink/Logic and Bit Operations/Bitwise Operator  logicop=AND  UseBitMask=on  BitMask=8  BitMaskRealWorld=Stored Integer
  Enable_Operation_Ctrl_O : Constant  Value=0  OutDataTypeStr=single
  Enable_Operation_Ctrl_S : ArithShift  BitShiftNumber=-3
  Enable_Operation_Ctrl_sat : Saturate  UpperLimit=1  LowerLimit=0
  Enable_Operation_Ctrl_st : Sum  Inputs=+-
  output1 : Outport
  wires:
  Enable_Operation_Ctrl/1 -> Enable_Operation_Ctrl_sat/1
  Enable_Operation_Ctrl_sat/1 -> Enable_Operation_Ctrl_st/1
  Enable_Operation_Ctrl_O/1 -> Enable_Operation_Ctrl_st/2
  Enable_Operation_Ctrl_st/1 -> Enable_Operation_Ctrl_D/1
  Enable_Operation_Ctrl_F/1 -> Enable_Operation_Ctrl_D/2
  Enable_Operation_Ctrl_D/1 -> Enable_Operation_CtrlRon/1
  Enable_Operation_CtrlRon/1 -> Enable_Operation_Ctrl_S/1
  Enable_Operation_Ctrl_S/1 -> Enable_Operation_Ctrl_1sat/1
  Enable_Operation_Ctrl_1sat/1 -> Enable_Operation_Ctrl_Convert1/1
  Enable_Operation_Ctrl_Convert1/1 -> Enable_Operation_Ctrl_L/1
  Enable_Operation_Ctrl_L/1 -> Enable_Operation_Ctrl_Convert/1
  Enable_Operation_Ctrl_Convert/1 -> output1/1

== system FSAC2021_V1_Running/CAN_SEND/Subsystem1/MOTEC_CONTROL/Enable_Voltage_Ctrl ==
  Enable_Voltage_Ctrl : Inport
  Enable_Voltage_CtrlRon : Rounding  Operator=round
  Enable_Voltage_Ctrl_1sat : Saturate  UpperLimit=2  LowerLimit=0
  Enable_Voltage_Ctrl_Convert : DataTypeConversion  OutDataTypeStr=uint8
  Enable_Voltage_Ctrl_Convert1 : DataTypeConversion  OutDataTypeStr=uint32
  Enable_Voltage_Ctrl_D : Product  Inputs=*/
  Enable_Voltage_Ctrl_F : Constant  OutDataTypeStr=single
  Enable_Voltage_Ctrl_L : simulink/Logic and Bit Operations/Bitwise Operator  logicop=AND  UseBitMask=on  BitMask=2  BitMaskRealWorld=Stored Integer
  Enable_Voltage_Ctrl_O : Constant  Value=0  OutDataTypeStr=single
  Enable_Voltage_Ctrl_S : ArithShift  BitShiftNumber=-1
  Enable_Voltage_Ctrl_sat : Saturate  UpperLimit=1  LowerLimit=0
  Enable_Voltage_Ctrl_st : Sum  Inputs=+-
  output1 : Outport
  wires:
  Enable_Voltage_Ctrl/1 -> Enable_Voltage_Ctrl_sat/1
  Enable_Voltage_Ctrl_sat/1 -> Enable_Voltage_Ctrl_st/1
  Enable_Voltage_Ctrl_O/1 -> Enable_Voltage_Ctrl_st/2
  Enable_Voltage_Ctrl_st/1 -> Enable_Voltage_Ctrl_D/1
  Enable_Voltage_Ctrl_F/1 -> Enable_Voltage_Ctrl_D/2
  Enable_Voltage_Ctrl_D/1 -> Enable_Voltage_CtrlRon/1
  Enable_Voltage_CtrlRon/1 -> Enable_Voltage_Ctrl_S/1
  Enable_Voltage_Ctrl_S/1 -> Enable_Voltage_Ctrl_1sat/1
  Enable_Voltage_Ctrl_1sat/1 -> Enable_Voltage_Ctrl_Convert1/1
  Enable_Voltage_Ctrl_Convert1/1 -> Enable_Voltage_Ctrl_L/1
  Enable_Voltage_Ctrl_L/1 -> Enable_Voltage_Ctrl_Convert/1
  Enable_Voltage_Ctrl_Convert/1 -> output1/1

== system FSAC2021_V1_Running/CAN_SEND/Subsystem1/MOTEC_CONTROL/Fault_Reset ==
  Fault_Reset : Inport
  Fault_ResetRon : Rounding  Operator=round
  Fault_Reset_1sat : Saturate  UpperLimit=128  LowerLimit=0
  Fault_Reset_Convert : DataTypeConversion  OutDataTypeStr=uint8
  Fault_Reset_Convert1 : DataTypeConversion  OutDataTypeStr=uint32
  Fault_Reset_D : Product  Inputs=*/
  Fault_Reset_F : Constant  OutDataTypeStr=single
  Fault_Reset_L : simulink/Logic and Bit Operations/Bitwise Operator  logicop=AND  UseBitMask=on  BitMask=128  BitMaskRealWorld=Stored Integer
  Fault_Reset_O : Constant  Value=0  OutDataTypeStr=single
  Fault_Reset_S : ArithShift  BitShiftNumber=-7
  Fault_Reset_sat : Saturate  UpperLimit=1  LowerLimit=0
  Fault_Reset_st : Sum  Inputs=+-
  output1 : Outport
  wires:
  Fault_Reset/1 -> Fault_Reset_sat/1
  Fault_Reset_sat/1 -> Fault_Reset_st/1
  Fault_Reset_O/1 -> Fault_Reset_st/2
  Fault_Reset_st/1 -> Fault_Reset_D/1
  Fault_Reset_F/1 -> Fault_Reset_D/2
  Fault_Reset_D/1 -> Fault_ResetRon/1
  Fault_ResetRon/1 -> Fault_Reset_S/1
  Fault_Reset_S/1 -> Fault_Reset_1sat/1
  Fault_Reset_1sat/1 -> Fault_Reset_Convert1/1
  Fault_Reset_Convert1/1 -> Fault_Reset_L/1
  Fault_Reset_L/1 -> Fault_Reset_Convert/1
  Fault_Reset_Convert/1 -> output1/1

== system FSAC2021_V1_Running/CAN_SEND/Subsystem1/MOTEC_CONTROL/Halt_Ctrl ==
  Halt_Ctrl : Inport
  Halt_CtrlRon : Rounding  Operator=round
  Halt_Ctrl_1sat : Saturate  UpperLimit=1  LowerLimit=0
  Halt_Ctrl_Convert : DataTypeConversion  OutDataTypeStr=uint8
  Halt_Ctrl_Convert1 : DataTypeConversion  OutDataTypeStr=uint32
  Halt_Ctrl_D : Product  Inputs=*/
  Halt_Ctrl_F : Constant  OutDataTypeStr=single
  Halt_Ctrl_L : simulink/Logic and Bit Operations/Bitwise Operator  logicop=AND  UseBitMask=on  BitMask=1  BitMaskRealWorld=Stored Integer
  Halt_Ctrl_O : Constant  Value=0  OutDataTypeStr=single
  Halt_Ctrl_S : ArithShift
  Halt_Ctrl_sat : Saturate  UpperLimit=1  LowerLimit=0
  Halt_Ctrl_st : Sum  Inputs=+-
  output2 : Outport
  wires:
  Halt_Ctrl/1 -> Halt_Ctrl_sat/1
  Halt_Ctrl_sat/1 -> Halt_Ctrl_st/1
  Halt_Ctrl_O/1 -> Halt_Ctrl_st/2
  Halt_Ctrl_st/1 -> Halt_Ctrl_D/1
  Halt_Ctrl_F/1 -> Halt_Ctrl_D/2
  Halt_Ctrl_D/1 -> Halt_CtrlRon/1
  Halt_CtrlRon/1 -> Halt_Ctrl_S/1
  Halt_Ctrl_S/1 -> Halt_Ctrl_1sat/1
  Halt_Ctrl_1sat/1 -> Halt_Ctrl_Convert1/1
  Halt_Ctrl_Convert1/1 -> Halt_Ctrl_L/1
  Halt_Ctrl_L/1 -> Halt_Ctrl_Convert/1
  Halt_Ctrl_Convert/1 -> output2/1

== system FSAC2021_V1_Running/CAN_SEND/Subsystem1/MOTEC_CONTROL/New_Pos_Set ==
  New_Pos_Set : Inport
  New_Pos_SetRon : Rounding  Operator=round
  New_Pos_Set_1sat : Saturate  UpperLimit=16  LowerLimit=0
  New_Pos_Set_Convert : DataTypeConversion  OutDataTypeStr=uint8
  New_Pos_Set_Convert1 : DataTypeConversion  OutDataTypeStr=uint32
  New_Pos_Set_D : Product  Inputs=*/
  New_Pos_Set_F : Constant  OutDataTypeStr=single
  New_Pos_Set_L : simulink/Logic and Bit Operations/Bitwise Operator  logicop=AND  UseBitMask=on  BitMask=16  BitMaskRealWorld=Stored Integer
  New_Pos_Set_O : Constant  Value=0  OutDataTypeStr=single
  New_Pos_Set_S : ArithShift  BitShiftNumber=-4
  New_Pos_Set_sat : Saturate  UpperLimit=1  LowerLimit=0
  New_Pos_Set_st : Sum  Inputs=+-
  output1 : Outport
  wires:
  New_Pos_Set/1 -> New_Pos_Set_sat/1
  New_Pos_Set_sat/1 -> New_Pos_Set_st/1
  New_Pos_Set_O/1 -> New_Pos_Set_st/2
  New_Pos_Set_st/1 -> New_Pos_Set_D/1
  New_Pos_Set_F/1 -> New_Pos_Set_D/2
  New_Pos_Set_D/1 -> New_Pos_SetRon/1
  New_Pos_SetRon/1 -> New_Pos_Set_S/1
  New_Pos_Set_S/1 -> New_Pos_Set_1sat/1
  New_Pos_Set_1sat/1 -> New_Pos_Set_Convert1/1
  New_Pos_Set_Convert1/1 -> New_Pos_Set_L/1
  New_Pos_Set_L/1 -> New_Pos_Set_Convert/1
  New_Pos_Set_Convert/1 -> output1/1

== system FSAC2021_V1_Running/CAN_SEND/Subsystem1/MOTEC_CONTROL/Position_set ==
  Position_set : Inport
  Position_setABS : Abs
  Position_setBitCov : DataTypeConversion  OutDataTypeStr=uint32
  Position_setBitCov1 : DataTypeConversion  OutDataTypeStr=uint32
  Position_setBitCov2 : DataTypeConversion  OutDataTypeStr=uint8
  Position_setCOV : DataTypeConversion  OutDataTypeStr=uint8
  Position_setCOV1 : DataTypeConversion  OutDataTypeStr=uint8
  Position_setCOV2 : DataTypeConversion  OutDataTypeStr=uint8
  Position_setCS : ArithShift  BitShiftNumber=-32
  Position_setConS : Constant  OutDataTypeStr=single
  Position_setCosR : Constant  Value=0  OutDataTypeStr=uint8
  Position_setROP : RelationalOperator  Operator=<  OutDataTypeStr=boolean
  Position_setRon : Rounding  Operator=round
  Position_setSW : Switch  Criteria=u2 ~= 0
  Position_set_1sat : Saturate  UpperLimit=4294967296  LowerLimit=0
  Position_set_And : simulink/Logic and Bit Operations/Bitwise Operator  logicop=AND  UseBitMask=off  NumInputPorts=2  BitMask=bin2dec('11011001')  BitMaskRealWorld=Stored Integer
  Position_set_And1 : simulink/Logic and Bit Operations/Bitwise Operator  logicop=AND  UseBitMask=off  NumInputPorts=2  BitMask=bin2dec('11011001')  BitMaskRealWorld=Stored Integer
  Position_set_And1_C : Constant  Value=65535
  Position_set_And2 : simulink/Logic and Bit Operations/Bitwise Operator  logicop=AND  UseBitMask=off  NumInputPorts=2  BitMask=bin2dec('11011001')  BitMaskRealWorld=Stored Integer
  Position_set_And2_C : Constant  Value=255  OutDataTypeStr=uint32
  Position_set_And_C : Constant  Value=16777215
  Position_set_Convert : DataTypeConversion  OutDataTypeStr=uint32
  Position_set_D{,1..3} (4 alike) : Product  Inputs=*/
  Position_set_F : Constant  Value=0.00144  OutDataTypeStr=single
  Position_set_L : simulink/Logic and Bit Operations/Bitwise Operator  logicop=AND  UseBitMask=on  BitMask=4294967295  BitMaskRealWorld=Stored Integer
  Position_set_O : Constant  Value=0  OutDataTypeStr=single
  Position_set_S : ArithShift
  Position_set_sat : Saturate  UpperLimit=3865470.5646  LowerLimit=-3865470.5664
  Position_set_st : Sum  Inputs=+-
  Position_setoutput4_C : Constant  Value=256
  Position_setoutput5_C : Constant  Value=65536
  Position_setoutput6_C : Constant  Value=16777216
  Position_setsubcon : Sum  Inputs=+-
  output3 : Outport
  output4 : Outport  Port=2
  output5 : Outport  Port=3
  output6 : Outport  Port=4
  wires:
  Position_set/1 -> Position_set_sat/1
  Position_set_sat/1 -> Position_set_st/1
  Position_set_O/1 -> Position_set_st/2
  Position_set_st/1 -> Position_set_D/1
  Position_set_F/1 -> Position_set_D/2
  Position_set_D/1 -> Position_setRon/1
  Position_setRon/1 -> Position_setROP/1, Position_setABS/1, Position_setSW/3
  Position_setCosR/1 -> Position_setROP/2
  Position_setConS/1 -> Position_setCS/1
  Position_setCS/1 -> Position_setsubcon/1
  Position_setABS/1 -> Position_setsubcon/2
  Position_setsubcon/1 -> Position_setSW/1
  Position_setROP/1 -> Position_setSW/2
  Position_setSW/1 -> Position_set_S/1
  Position_set_S/1 -> Position_set_1sat/1
  Position_set_1sat/1 -> Position_set_Convert/1
  Position_set_Convert/1 -> Position_set_L/1
  Position_set_L/1 -> Position_set_And1/1, Position_set_And2/1, Position_set_And/1, Position_set_D1/1
  Position_setoutput6_C/1 -> Position_set_D1/2
  Position_set_D1/1 -> Position_setCOV/1
  Position_setCOV/1 -> output6/1
  Position_set_And_C/1 -> Position_setBitCov/1
  Position_setBitCov/1 -> Position_set_And/2
  Position_set_And/1 -> Position_set_D2/1
  Position_setoutput5_C/1 -> Position_set_D2/2
  Position_set_D2/1 -> Position_setCOV1/1
  Position_setCOV1/1 -> output5/1
  Position_set_And1_C/1 -> Position_setBitCov1/1
  Position_setBitCov1/1 -> Position_set_And1/2
  Position_set_And1/1 -> Position_set_D3/1
  Position_setoutput4_C/1 -> Position_set_D3/2
  Position_set_D3/1 -> Position_setCOV2/1
  Position_setCOV2/1 -> output4/1
  Position_set_And2_C/1 -> Position_set_And2/2
  Position_set_And2/1 -> Position_setBitCov2/1
  Position_setBitCov2/1 -> output3/1

== system FSAC2021_V1_Running/CAN_SEND/Subsystem1/MOTEC_CONTROL/Quick_Stop_Ctrl ==
  Quick_Stop_Ctrl : Inport
  Quick_Stop_CtrlRon : Rounding  Operator=round
  Quick_Stop_Ctrl_1sat : Saturate  UpperLimit=4  LowerLimit=0
  Quick_Stop_Ctrl_Convert : DataTypeConversion  OutDataTypeStr=uint8
  Quick_Stop_Ctrl_Convert1 : DataTypeConversion  OutDataTypeStr=uint32
  Quick_Stop_Ctrl_D : Product  Inputs=*/
  Quick_Stop_Ctrl_F : Constant  OutDataTypeStr=single
  Quick_Stop_Ctrl_L : simulink/Logic and Bit Operations/Bitwise Operator  logicop=AND  UseBitMask=on  BitMask=4  BitMaskRealWorld=Stored Integer
  Quick_Stop_Ctrl_O : Constant  Value=0  OutDataTypeStr=single
  Quick_Stop_Ctrl_S : ArithShift  BitShiftNumber=-2
  Quick_Stop_Ctrl_sat : Saturate  UpperLimit=1  LowerLimit=0
  Quick_Stop_Ctrl_st : Sum  Inputs=+-
  output1 : Outport
  wires:
  Quick_Stop_Ctrl/1 -> Quick_Stop_Ctrl_sat/1
  Quick_Stop_Ctrl_sat/1 -> Quick_Stop_Ctrl_st/1
  Quick_Stop_Ctrl_O/1 -> Quick_Stop_Ctrl_st/2
  Quick_Stop_Ctrl_st/1 -> Quick_Stop_Ctrl_D/1
  Quick_Stop_Ctrl_F/1 -> Quick_Stop_Ctrl_D/2
  Quick_Stop_Ctrl_D/1 -> Quick_Stop_CtrlRon/1
  Quick_Stop_CtrlRon/1 -> Quick_Stop_Ctrl_S/1
  Quick_Stop_Ctrl_S/1 -> Quick_Stop_Ctrl_1sat/1
  Quick_Stop_Ctrl_1sat/1 -> Quick_Stop_Ctrl_Convert1/1
  Quick_Stop_Ctrl_Convert1/1 -> Quick_Stop_Ctrl_L/1
  Quick_Stop_Ctrl_L/1 -> Quick_Stop_Ctrl_Convert/1
  Quick_Stop_Ctrl_Convert/1 -> output1/1

== system FSAC2021_V1_Running/CAN_SEND/Subsystem1/MOTEC_CONTROL/Switch_On_Ctrl ==
  Switch_On_Ctrl : Inport
  Switch_On_CtrlRon : Rounding  Operator=round
  Switch_On_Ctrl_1sat : Saturate  UpperLimit=1  LowerLimit=0
  Switch_On_Ctrl_Convert : DataTypeConversion  OutDataTypeStr=uint8
  Switch_On_Ctrl_Convert1 : DataTypeConversion  OutDataTypeStr=uint32
  Switch_On_Ctrl_D : Product  Inputs=*/
  Switch_On_Ctrl_F : Constant  OutDataTypeStr=single
  Switch_On_Ctrl_L : simulink/Logic and Bit Operations/Bitwise Operator  logicop=AND  UseBitMask=on  BitMask=1  BitMaskRealWorld=Stored Integer
  Switch_On_Ctrl_O : Constant  Value=0  OutDataTypeStr=single
  Switch_On_Ctrl_S : ArithShift
  Switch_On_Ctrl_sat : Saturate  UpperLimit=1  LowerLimit=0
  Switch_On_Ctrl_st : Sum  Inputs=+-
  output1 : Outport
  wires:
  Switch_On_Ctrl/1 -> Switch_On_Ctrl_sat/1
  Switch_On_Ctrl_sat/1 -> Switch_On_Ctrl_st/1
  Switch_On_Ctrl_O/1 -> Switch_On_Ctrl_st/2
  Switch_On_Ctrl_st/1 -> Switch_On_Ctrl_D/1
  Switch_On_Ctrl_F/1 -> Switch_On_Ctrl_D/2
  Switch_On_Ctrl_D/1 -> Switch_On_CtrlRon/1
  Switch_On_CtrlRon/1 -> Switch_On_Ctrl_S/1
  Switch_On_Ctrl_S/1 -> Switch_On_Ctrl_1sat/1
  Switch_On_Ctrl_1sat/1 -> Switch_On_Ctrl_Convert1/1
  Switch_On_Ctrl_Convert1/1 -> Switch_On_Ctrl_L/1
  Switch_On_Ctrl_L/1 -> Switch_On_Ctrl_Convert/1
  Switch_On_Ctrl_Convert/1 -> output1/1
